simulink model "nomoto2"  (R2017b)
settings: Solver=VariableStepAuto  StartTime=0.0  StopTime=tstop  RelTol=1e-3
values from neighbouring files (symbols this model uses):
  dc = 3*deg2rad    (= 0.0523598775598)    [TTK4190_A3_task1_2.m]    (also in model_analysis.m = dc_list(i); sim_nomoto2.m = delta_c; sysID.m = dc_list(i))
  K2 = 0.00466/dc    (= 0.088999444177)    [TTK4190_A3_task1_2.m]    (also in TTK4190_A3_task1_3.m = -0.04)
  T1 = 250    [TTK4190_A3_task1_2.m]    (also in TTK4190_A3_task1_3.m = 204; model_analysis.m = x(1))
  T2 = 325    [TTK4190_A3_task1_2.m]    (also in TTK4190_A3_task1_3.m = 224; model_analysis.m = x(2))
  T3 = 490    [TTK4190_A3_task1_2.m]    (also in TTK4190_A3_task1_3.m = 423; model_analysis.m = x(3))
  tsamp = 10    [TTK4190_A3_task1_2.m]    (also in TTK4190_A3_task1_3.m; model_analysis.m = 35; sim_nomoto2.m = tsamp; sysID.m = 100)
  x = lsqcurvefit(F4, x0, t, r,[],[],OPT)    [model_analysis.m]
settings Model: Creator=Kjetil  LastModifiedBy=Kjetil

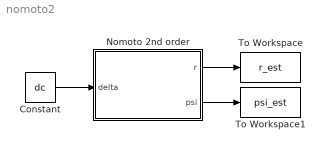
== system nomoto2 ==
  Constant : Constant  Value=dc
  Nomoto 2nd order : Subsystem
  To Workspace : ToWorkspace  VariableName=r_est  SampleTime=tsamp
  To Workspace1 : ToWorkspace  VariableName=psi_est  SampleTime=tsamp
  wires:
  Nomoto 2nd order/1(r) -> To Workspace/1
  Nomoto 2nd order/2(psi) -> To Workspace1/1
  Constant/1 -> Nomoto 2nd order/1(delta)

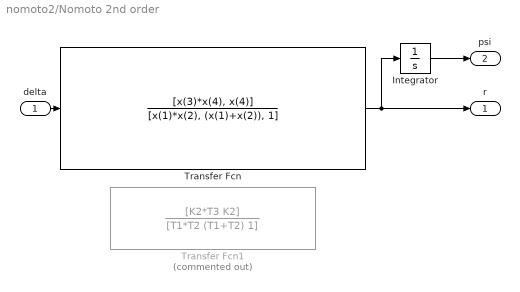
== system nomoto2/Nomoto 2nd order ==
  delta : Inport
  Integrator : Integrator
  Transfer Fcn : TransferFcn  Numerator=[x(3)*x(4), x(4)]  Denominator=[x(1)*x(2), (x(1)+x(2)), 1]
  Transfer Fcn1 : TransferFcn  Commented=on  Numerator=[K2*T3 K2]  Denominator=[T1*T2 (T1+T2) 1]
  r : Outport
  psi : Outport  Port=2
  wires:
  Integrator/1 -> psi/1
  delta/1 -> Transfer Fcn/1
  Transfer Fcn/1 -> r/1, Integrator/1
